simulink subsystem "ConfiguredSimscapePlantModels"  (R2022b)
settings: Solver=VariableStepAuto  StartTime=0.0  StopTime=10.0  RelTol=1e-3
undefined symbols (not defined in the file): AxlFL, AxlFR, AxlRL, AxlRR, EM1, EM2, PlntDCDCVoltInit, PlntDiffrntl2Axl1Damp, PlntDiffrntl2CarrDamp, PlntDiffrntl2Eff, PlntDiffrntl2PwrThresh, PlntDiffrntlAxl1Damp, PlntDiffrntlCarrDamp, PlntDiffrntlEff, PlntDiffrntlPwrThresh, PlntTrnsfrCaseAxlSpdLock, PlntTrnsfrCaseTrqSplitRatio
libraries: fl_lib x14, nesl_utility_internal x10, sdl_lib x5, nesl_utility x1
(part 1 of 2)
settings Model: ModifiedByFormat=The MathWorks, Inc.  Creator=The MathWorks, Inc.  LastModifiedBy=The MathWorks, Inc.
settings SolverCC: MaxZcPerStep=1
settings DebuggingCC: UnconnectedInputMsg=warning  UnconnectedOutputMsg=warning  UnconnectedLineMsg=warning
settings ModelReferenceCC: EnableRefExpFcnMdlSchedulingChecks=on
settings RTWCC: DLArmComputeVersion=19.05

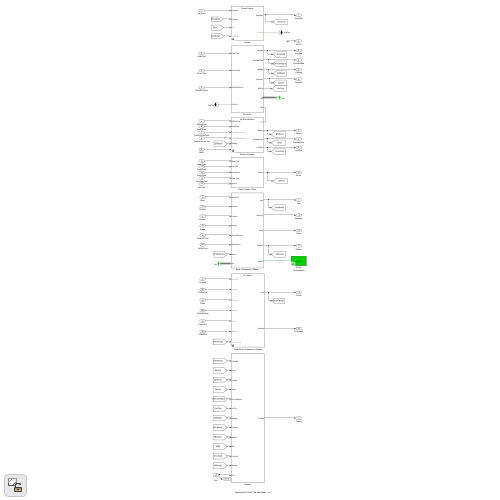
[thumbnail: Simulink's stored preview of the top-level diagram]
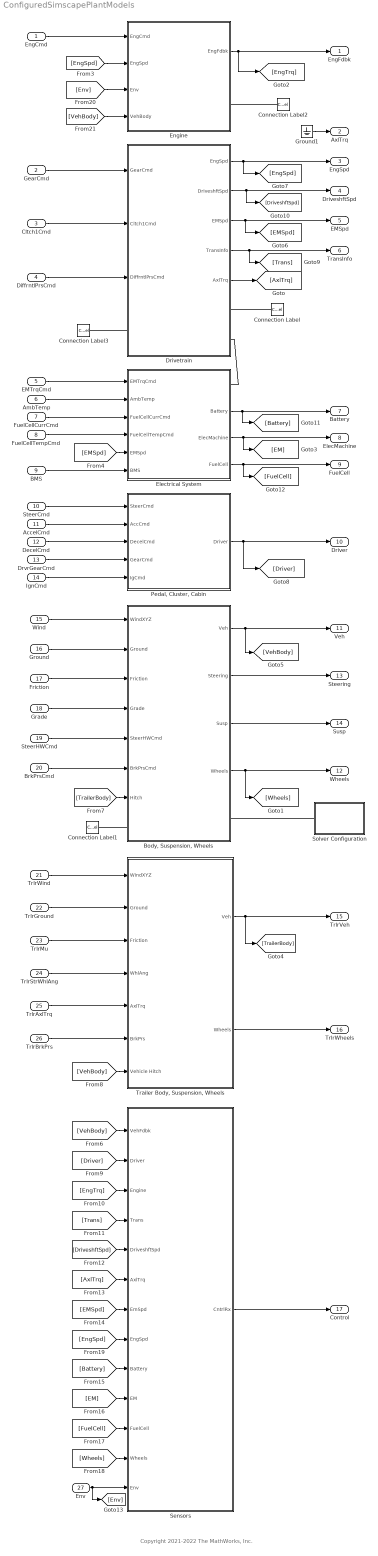
== system ConfiguredSimscapePlantModels ==
  note: Copyright 2021-2022 The MathWorks, Inc.
  EngCmd : Inport
  GearCmd : Inport  Port=2
  Cltch1Cmd : Inport  Port=3
  DiffrntlPrsCmd : Inport  Port=4
  EMTrqCmd : Inport  Port=5
  AmbTemp : Inport  Port=6
  FuelCellCurrCmd : Inport  Port=7
  FuelCellTempCmd : Inport  Port=8
  BMS : Inport  Port=9
  SteerCmd : Inport  Port=10
  AccelCmd : Inport  Port=11
  DecelCmd : Inport  Port=12
  DrvrGearCmd : Inport  Port=13
  IgnCmd : Inport  Port=14
  Wind : Inport  Port=15
  Ground : Inport  Port=16
  Friction : Inport  Port=17
  Grade : Inport  Port=18
  SteerHWCmd : Inport  Port=19
  BrkPrsCmd : Inport  Port=20
  TrlrWind : Inport  Port=21
  TrlrGround : Inport  Port=22
  TrlrMu : Inport  Port=23
  TrlrStrWhlAng : Inport  Port=24
  TrlrAxlTrq : Inport  Port=25
  TrlrBrkPrs : Inport  Port=26
  " Env" : Inport  Port=27
  "Body, Suspension, Wheels" : Subsystem  VariantControl=Longitudinal Vehicle Dynamics
  Connection Label : ConnectionLabel  Label=Axl
  Connection Label1 : ConnectionLabel  Label=Axl
  Connection Label2 : ConnectionLabel  Label=EngTrq
  Connection Label3 : ConnectionLabel  Label=EngTrq
  Drivetrain : Subsystem
  Electrical System : Subsystem  Variant=on  VariantControlMode=label  VariantControl=Choice  LabelModeActiveChoice=Electrical System 1EM
      settings: PortSchema="{\"entries\":[{\"content\":{\"sides\":[{\"content\":{\"connectorIds\":[\"In1\",\"In2\",\"In3\",\"In4\",\"In5\",\"In6\"]},\"type\":\"ConnectorPlacement.EquallySpacedRectSide\",\"uuid\":\"168fda7d-02fd-4045-80e4-d70d0b749a9c\"},{\"content\":{\"connectorIds\":[\"RConn1\",\"Out1\",\"Out2\",\"Out3\"],\"side\":\"RIGHT\"},\"type\":\"ConnectorPlacement.EquallySpacedRectSide\",\"uuid\":\"a7e9bf4a-b9ce-46d6-8afc-0075c6e03a0c\"},{\"content\":{\"connectorIds\":[],\"side\":\"TOP\"},\"type\":\"ConnectorPlacement.EquallySpacedRectSide\",\"uuid\":\"81c60468-d7ed-4851-a727-3a9a5b008640\"}]},\"type\":\"ConnectorPlacement.EquallySpacedConnector\",\"uuid\":\"8c7c8f28-264e-479c-b2d0-01b49dca4966\"}],\"packageUris\":[\"http://schema.mathworks.com/mf0/Connector/R2020b\"],\"version\":\"1.0\"}"
  Engine : Subsystem  Variant=on  VariantControlMode=label  LabelModeActiveChoice=No Engine
  Ground1 : Ground
  "Pedal, Cluster, Cabin" : Subsystem
  Sensors : Subsystem
  Solver Configuration : Subsystem  Variant=on  VariantControlMode=label  VariantControl=Choice  LabelModeActiveChoice=Solver Configuration
  "Trailer Body, Suspension, Wheels" : Subsystem  Variant=on  VariantControlMode=label  LabelModeActiveChoice=No Trailer
  EngFdbk : Outport
  AxlTrq : Outport  Port=2
  EngSpd : Outport  Port=3
  DriveshftSpd : Outport  Port=4
  EMSpd : Outport  Port=5
  TransInfo : Outport  Port=6
  Battery : Outport  Port=7
  ElecMachine : Outport  Port=8
  FuelCell : Outport  Port=9
  Driver : Outport  Port=10
  Veh : Outport  Port=11
  Wheels : Outport  Port=12
  Steering : Outport  Port=13
  Susp : Outport  Port=14
  TrlrVeh : Outport  Port=15
  TrlrWheels : Outport  Port=16
  Control : Outport  Port=17
  wires:
  Drivetrain/4(TransInfo) -> [Trans], TransInfo/1
  EngCmd/1 -> Engine/1(EngCmd)
  Electrical System/3(FuelCell) -> FuelCell/1, [FuelCell]
  Electrical System/1(Battery) -> Battery/1, [Battery]
  TrlrGround/1 -> "Trailer Body, Suspension, Wheels"/2(Ground)
  Wind/1 -> "Body, Suspension, Wheels"/1(WindXYZ)
  TrlrAxlTrq/1 -> "Trailer Body, Suspension, Wheels"/5(AxlTrq)
  EMTrqCmd/1 -> Electrical System/1(EMTrqCmd)
  DiffrntlPrsCmd/1 -> Drivetrain/3(DiffrntlPrsCmd)
  TrlrMu/1 -> "Trailer Body, Suspension, Wheels"/3(Friction)
  Friction/1 -> "Body, Suspension, Wheels"/3(Friction)
  SteerHWCmd/1 -> "Body, Suspension, Wheels"/5(SteerHWCmd)
  [EMSpd] -> Electrical System/5(EMSpd)
  Ground/1 -> "Body, Suspension, Wheels"/2(Ground)
  AmbTemp/1 -> Electrical System/2(AmbTemp)
  SteerCmd/1 -> "Pedal, Cluster, Cabin"/1(SteerCmd)
  TrlrBrkPrs/1 -> "Trailer Body, Suspension, Wheels"/6(BrkPrs)
  Drivetrain/2(DriveshftSpd) -> [DriveshftSpd], DriveshftSpd/1
  "Body, Suspension, Wheels"/1(Veh) -> [VehBody], Veh/1
  Engine/1(EngFdbk) -> [EngTrq], EngFdbk/1
  BrkPrsCmd/1 -> "Body, Suspension, Wheels"/6(BrkPrsCmd)
  Cltch1Cmd/1 -> Drivetrain/2(Cltch1Cmd)
  TrlrWind/1 -> "Trailer Body, Suspension, Wheels"/1(WindXYZ)
  TrlrStrWhlAng/1 -> "Trailer Body, Suspension, Wheels"/4(WhlAng)
  [VehBody] -> "Trailer Body, Suspension, Wheels"/7(Vehicle Hitch)
  "Trailer Body, Suspension, Wheels"/2(Wheels) -> TrlrWheels/1
  Electrical System/2(ElecMachine) -> [EM], ElecMachine/1
  [TrailerBody] -> "Body, Suspension, Wheels"/7(Hitch)
  DecelCmd/1 -> "Pedal, Cluster, Cabin"/3(DecelCmd)
  DrvrGearCmd/1 -> "Pedal, Cluster, Cabin"/4(GearCmd)
  Drivetrain/3(EMSpd) -> [EMSpd], EMSpd/1
  IgnCmd/1 -> "Pedal, Cluster, Cabin"/5(IgCmd)
  FuelCellTempCmd/1 -> Electrical System/4(FuelCellTempCmd)
  "Body, Suspension, Wheels"/2(Steering) -> Steering/1
  GearCmd/1 -> Drivetrain/1(GearCmd)
  "Body, Suspension, Wheels"/4(Wheels) -> [Wheels], Wheels/1
  "Trailer Body, Suspension, Wheels"/1(Veh) -> TrlrVeh/1, [TrailerBody]
  FuelCellCurrCmd/1 -> Electrical System/3(FuelCellCurrCmd)
  AccelCmd/1 -> "Pedal, Cluster, Cabin"/2(AccCmd)
  Drivetrain/1(EngSpd) -> EngSpd/1, [EngSpd]
  [VehBody] -> Sensors/1(VehFdbk)
  "Pedal, Cluster, Cabin"/1(Driver) -> Driver/1, [Driver]
  [Driver] -> Sensors/2(Driver)
  [EngTrq] -> Sensors/3(Engine)
  [Trans] -> Sensors/4(Trans)
  [DriveshftSpd] -> Sensors/5(DriveshftSpd)
  [AxlTrq] -> Sensors/6(AxlTrq)
  [EMSpd] -> Sensors/7(EmSpd)
  [Battery] -> Sensors/9(Battery)
  [EM] -> Sensors/10(EM)
  [FuelCell] -> Sensors/11(FuelCell)
  [Wheels] -> Sensors/12(Wheels)
  Sensors/1(CntrlRx) -> Control/1
  " Env"/1 -> Sensors/13(Env), [Env]
  [EngSpd] -> Sensors/8(EngSpd)
  [Env] -> Engine/3(Env)
  [VehBody] -> Engine/4(VehBody)
  [EngSpd] -> Engine/2(EngSpd)
  "Body, Suspension, Wheels"/3(Susp) -> Susp/1
  Grade/1 -> "Body, Suspension, Wheels"/4(Grade)
  Ground1/1 -> AxlTrq/1
  Drivetrain/5(AxlTrq) -> [AxlTrq]
  BMS/1 -> Electrical System/6(BMS)
  connections:
  Connection Label/LConn1 -- Drivetrain/RConn1
  "Body, Suspension, Wheels"/LConn1 -- Connection Label1/LConn1
  Electrical System/RConn1 -- Drivetrain/RConn2
  Drivetrain/LConn1 -- Connection Label3/LConn1
  Connection Label2/LConn1 -- Engine/RConn1
  Solver Configuration/RConn1 -- "Body, Suspension, Wheels"/RConn1

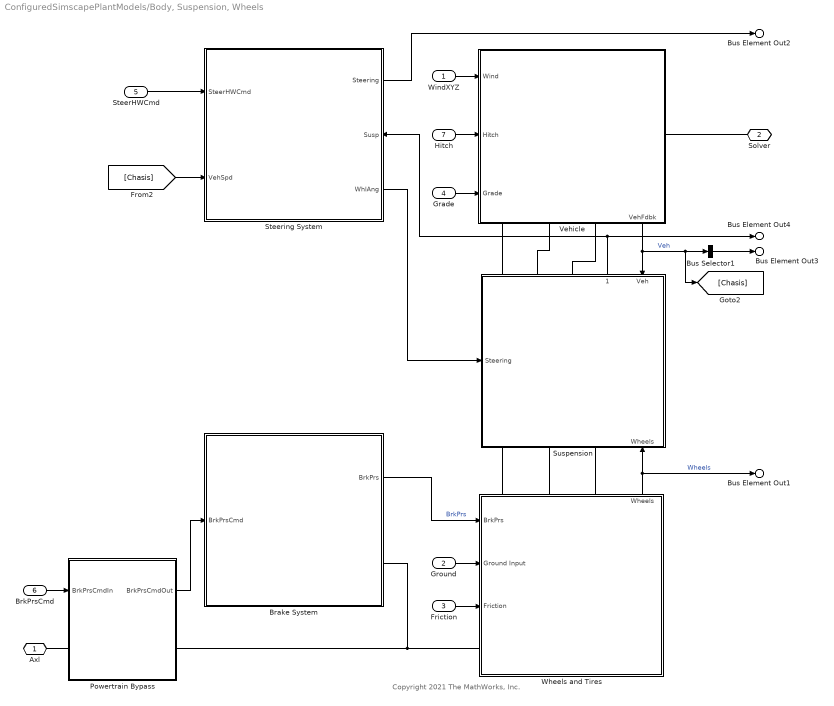
== system ConfiguredSimscapePlantModels/Body, Suspension, Wheels ==
  note: Copyright 2021 The MathWorks, Inc.
  WindXYZ : Inport  Unit=m/s  PortDimensions=3
  Ground : Inport  Port=2  Unit=m  PortDimensions=4
  Friction : Inport  Port=3  Unit=1  PortDimensions=4
  Grade : Inport  Port=4  Unit=deg  PortDimensions=1
  SteerHWCmd : Inport  Port=5  Unit=rad
  BrkPrsCmd : Inport  Port=6  PortDimensions=4
  Hitch : Inport  Port=7
  Brake System : Subsystem  Variant=on  VariantControlMode=label  VariantControl=Choice  LabelModeActiveChoice=Braking Hydraulics and Disc Brakes
      mask Display: disp('Brake System');
  Bus Selector1 : BusSelector  OutputSignals=InertFrm,BdyFrm  OutputAsBus=on
  Powertrain Bypass : Subsystem  Variant=on  VariantControlMode=label  VariantControl=Choice  LabelModeActiveChoice=Pass Through
  Steering System : Subsystem  Variant=on  VariantControlMode=label  VariantControl=0  LabelModeActiveChoice=No Steering
      settings: PortSchema="{\"entries\":[{\"content\":{\"sides\":[{\"content\":{\"connectorIds\":[\"In1\",\"In2\"]},\"type\":\"ConnectorPlacement.EquallySpacedRectSide\",\"uuid\":\"f4eae9a1-ee72-4894-9c3f-d81ee40fba89\"},{\"content\":{\"connectorIds\":[\"Out1\",\"In3\",\"Out2\"],\"side\":\"RIGHT\"},\"type\":\"ConnectorPlacement.EquallySpacedRectSide\",\"uuid\":\"c62a78d9-dc5d-4f96-a554-c82d7fa22a9e\"},{\"content\":{\"connectorIds\":[],\"side\":\"TOP\"},\"type\":\"ConnectorPlacement.EquallySpacedRectSide\",\"uuid\":\"38f3851a-1d1e-4a2b-8c09-8e5c8dcc7723\"}]},\"type\":\"ConnectorPlacement.EquallySpacedConnector\",\"uuid\":\"9f269846-92fa-4948-bc2b-71154f41fdde\"}],\"packageUris\":[\"http://schema.mathworks.com/mf0/Connector/R2020b\"],\"version\":\"1.0\"}"
      mask Display: disp('Steering System');
  Suspension : Subsystem  Variant=on  VariantControlMode=label  VariantControl=Choice  LabelModeActiveChoice=No Suspension
      settings: PortSchema="{\"entries\":[{\"content\":{\"sides\":[{\"content\":{\"connectorIds\":[\"In1\"]},\"type\":\"ConnectorPlacement.EquallySpacedRectSide\",\"uuid\":\"0a9265e3-f55e-4b74-9b74-681dc9522591\"},{\"content\":{\"connectorIds\":[],\"side\":\"RIGHT\"},\"type\":\"ConnectorPlacement.EquallySpacedRectSide\",\"uuid\":\"92df639a-7bc2-4e90-97ea-0cb216e2f16a\"},{\"content\":{\"connectorIds\":[\"LConn1\",\"LConn2\",\"LConn3\",\"Out1\",\"In2\"],\"side\":\"TOP\"},\"type\":\"ConnectorPlacement.EquallySpacedRectSide\",\"uuid\":\"2064b6cb-c7a8-4cfb-82de-a07750d990cb\"},{\"content\":{\"connectorIds\":[\"RConn1\",\"RConn2\",\"RConn3\",\"In3\"],\"side\":\"BOTTOM\"},\"type\":\"ConnectorPlacement.EquallySpacedRectSide\",\"uuid\":\"169bd4e6-c3fe-4e36-acea-c25875014463\"}]},\"type\":\"ConnectorPlacement.EquallySpacedConnector\",\"uuid\":\"e0b50182-0637-4594-80e7-4ddd0df85797\"}],\"packageUris\":[\"http://schema.mathworks.com/mf0/Connector/R2020b\"],\"version\":\"1.0\"}"
      mask Display: disp('Suspension');
  Vehicle : Subsystem  Variant=on  VariantControlMode=label  VariantControl=Choice  LabelModeActiveChoice=Vehicle Body 1DOF Longitudinal
      settings: PortSchema="{\"entries\":[{\"content\":{\"sides\":[{\"content\":{\"connectorIds\":[\"In1\",\"In2\",\"In3\"]},\"type\":\"ConnectorPlacement.EquallySpacedRectSide\",\"uuid\":\"0a9265e3-f55e-4b74-9b74-681dc9522591\"},{\"content\":{\"connectorIds\":[\"RConn1\"],\"side\":\"RIGHT\"},\"type\":\"ConnectorPlacement.EquallySpacedRectSide\",\"uuid\":\"92df639a-7bc2-4e90-97ea-0cb216e2f16a\"},{\"content\":{\"connectorIds\":[],\"side\":\"TOP\"},\"type\":\"ConnectorPlacement.EquallySpacedRectSide\",\"uuid\":\"2064b6cb-c7a8-4cfb-82de-a07750d990cb\"},{\"content\":{\"connectorIds\":[\"RConn2\",\"RConn3\",\"RConn4\",\"Out1\"],\"side\":\"BOTTOM\"},\"type\":\"ConnectorPlacement.EquallySpacedRectSide\",\"uuid\":\"2b34afca-0a88-43db-924f-6476183b84bd\"}]},\"type\":\"ConnectorPlacement.EquallySpacedConnector\",\"uuid\":\"e0b50182-0637-4594-80e7-4ddd0df85797\"}],\"packageUris\":[\"http://schema.mathworks.com/mf0/Connector/R2020b\"],\"version\":\"1.0\"}"
      mask Display: disp('Vehicle');
  Wheels and Tires : Subsystem  Variant=on  VariantControlMode=label  VariantControl=Choice  LabelModeActiveChoice=MF Tires Longitudinal
      settings: PortSchema="{\"entries\":[{\"content\":{\"sides\":[{\"content\":{\"connectorIds\":[\"In1\",\"In2\",\"In3\",\"LConn1\"]},\"type\":\"ConnectorPlacement.EquallySpacedRectSide\",\"uuid\":\"fdb4d4cd-d0c0-42d9-b073-775af31e96a1\"},{\"content\":{\"connectorIds\":[],\"side\":\"RIGHT\"},\"type\":\"ConnectorPlacement.EquallySpacedRectSide\",\"uuid\":\"04106ddf-9917-4cd4-b177-ae763d642686\"},{\"content\":{\"connectorIds\":[\"LConn2\",\"LConn3\",\"LConn4\",\"Out1\"],\"side\":\"TOP\"},\"type\":\"ConnectorPlacement.EquallySpacedRectSide\",\"uuid\":\"568bf95c-0e25-4c45-a134-c198357b75be\"}]},\"type\":\"ConnectorPlacement.EquallySpacedConnector\",\"uuid\":\"4f44df5e-0d14-43ea-934e-2abe86546e95\"}],\"packageUris\":[\"http://schema.mathworks.com/mf0/Connector/R2020b\"],\"version\":\"1.0\"}"
      mask Display: disp('Suspension');
  Axl : PMIOPort  Side=Left
  Solver : PMIOPort  Port=2  Side=Right
  Bus Element Out3 : Outport  PortName=Veh
  Bus Element Out2 : Outport  Port=2  PortName=Steering
  Bus Element Out4 : Outport  Port=3  PortName=Susp
  Bus Element Out1 : Outport  Port=4  PortName=Wheels
  wires:
  SteerHWCmd/1 -> Steering System/1(SteerHWCmd)
  Bus Selector1/1 -> Bus Element Out3/1
  WindXYZ/1 -> Vehicle/1(Wind)
  Brake System/1(BrkPrs) -> Wheels and Tires/1(BrkPrs)  "BrkPrs"
  Steering System/2(WhlAng) -> Suspension/1(Steering)
  Suspension/1(SuspChassis) -> Steering System/3(Susp), Bus Element Out4/1
  Powertrain Bypass/1(BrkPrsCmdOut) -> Brake System/1(BrkPrsCmd)
  Wheels and Tires/1(Wheels) -> Bus Element Out1/1, Suspension/3(Wheels)  "Wheels"
  Grade/1 -> Vehicle/3(Grade)
  Hitch/1 -> Vehicle/2(Hitch)
  Friction/1 -> Wheels and Tires/3(Friction)
  Steering System/1(Steering) -> Bus Element Out2/1
  [Chasis] -> Steering System/2(VehSpd)
  Ground/1 -> Wheels and Tires/2(Ground Input)
  Vehicle/1(VehFdbk) -> [Chasis], Bus Selector1/1, Suspension/2(Veh)  "Veh"
  BrkPrsCmd/1 -> Powertrain Bypass/1(BrkPrsCmdIn)
  connections:
  Brake System/RConn1 -- Powertrain Bypass/RConn1 -- Wheels and Tires/LConn1
  Vehicle/RConn2 -- Suspension/LConn1
  Vehicle/RConn3 -- Suspension/LConn2
  Vehicle/RConn4 -- Suspension/LConn3
  Wheels and Tires/LConn2 -- Suspension/RConn1
  Wheels and Tires/LConn3 -- Suspension/RConn2
  Wheels and Tires/LConn4 -- Suspension/RConn3
  Vehicle/RConn1 -- Solver/RConn1
  Axl/RConn1 -- Powertrain Bypass/LConn1

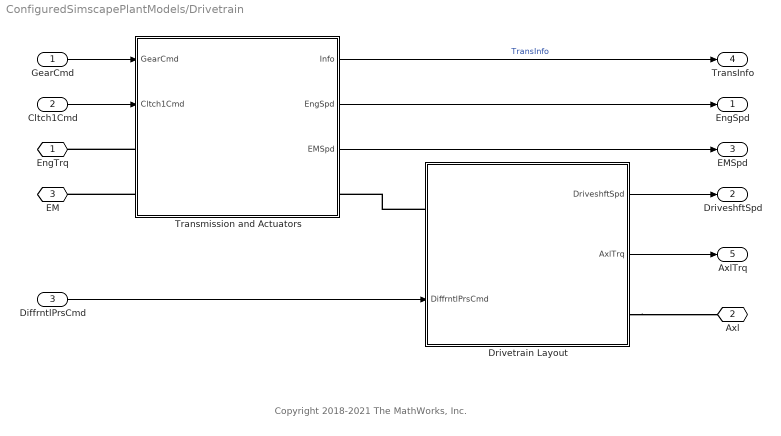
== system ConfiguredSimscapePlantModels/Drivetrain ==
  note: Copyright 2018-2021 The MathWorks, Inc.
  GearCmd : Inport
  Cltch1Cmd : Inport  Port=2
  DiffrntlPrsCmd : Inport  Port=3
  Drivetrain Layout : Subsystem  VariantControl=New
      settings: PortSchema="{\"entries\":[{\"content\":{\"sides\":[{\"content\":{\"connectorIds\":[\"LConn1\",\"In1\"]},\"type\":\"ConnectorPlacement.EquallySpacedRectSide\",\"uuid\":\"aca18566-8f68-4dbe-a1ea-7891e9b0f8a0\"},{\"content\":{\"connectorIds\":[\"Out1\",\"Out2\",\"RConn1\"],\"side\":\"RIGHT\"},\"type\":\"ConnectorPlacement.EquallySpacedRectSide\",\"uuid\":\"80817b32-8ae2-43ef-bc82-fae1c7a772cb\"},{\"content\":{\"connectorIds\":[],\"side\":\"TOP\"},\"type\":\"ConnectorPlacement.EquallySpacedRectSide\",\"uuid\":\"fadb27fa-7a73-4d3f-b69d-888e371ed2d5\"}]},\"type\":\"ConnectorPlacement.EquallySpacedConnector\",\"uuid\":\"7287b0c1-67df-44d5-bf90-b5b5a04fa161\"}],\"packageUris\":[\"http://schema.mathworks.com/mf0/Connector/R2020b\"],\"version\":\"1.0\"}"
  Transmission and Actuators : Subsystem  Variant=on  VariantControlMode=label  LabelModeActiveChoice=Electric Vehicle 1EM
  EngTrq : PMIOPort  Side=Left
  Axl : PMIOPort  Port=2  Side=Right
  EM : PMIOPort  Port=3  Side=Right
  EngSpd : Outport  Unit=rad/s  VectorParamsAs1DForOutWhenUnconnected=off
  DriveshftSpd : Outport  Port=2  VectorParamsAs1DForOutWhenUnconnected=off
  EMSpd : Outport  Port=3  Unit=rad/s  VectorParamsAs1DForOutWhenUnconnected=off
  TransInfo : Outport  Port=4  VectorParamsAs1DForOutWhenUnconnected=off
  AxlTrq : Outport  Port=5  VectorParamsAs1DForOutWhenUnconnected=off
  wires:
  Transmission and Actuators/1(Info) -> TransInfo/1  "TransInfo"
  DiffrntlPrsCmd/1 -> Drivetrain Layout/1(DiffrntlPrsCmd)
  Cltch1Cmd/1 -> Transmission and Actuators/2(Cltch1Cmd)
  Drivetrain Layout/1(DriveshftSpd) -> DriveshftSpd/1
  GearCmd/1 -> Transmission and Actuators/1(GearCmd)
  Transmission and Actuators/2(EngSpd) -> EngSpd/1
  Transmission and Actuators/3(EMSpd) -> EMSpd/1
  Drivetrain Layout/2(AxlTrq) -> AxlTrq/1
  connections:
  Transmission and Actuators/LConn2 -- EM/RConn1
  Drivetrain Layout/RConn1 -- Axl/RConn1
  Drivetrain Layout/LConn1 -- Transmission and Actuators/RConn1
  Transmission and Actuators/LConn1 -- EngTrq/RConn1

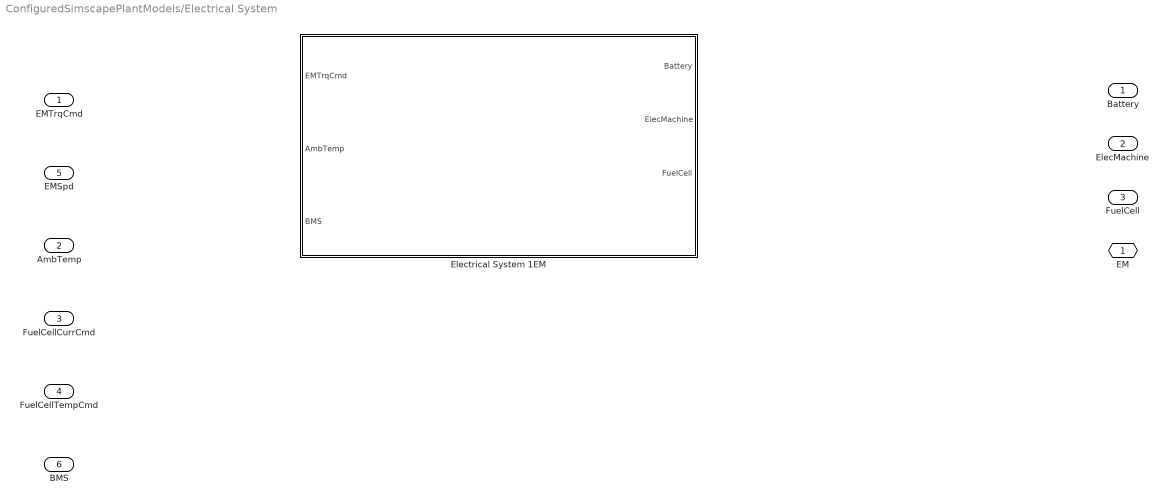
== system ConfiguredSimscapePlantModels/Electrical System ==
  EMTrqCmd : Inport
  AmbTemp : Inport  Port=2
  FuelCellCurrCmd : Inport  Port=3
  FuelCellTempCmd : Inport  Port=4
  EMSpd : Inport  Port=5
  BMS : Inport  Port=6
  Electrical System 1EM : Subsystem  VariantControl=Electrical System 1EM
  EM : PMIOPort  Side=Right
  Battery : Outport
  ElecMachine : Outport  Port=2
  FuelCell : Outport  Port=3

== system ConfiguredSimscapePlantModels/Engine ==
  EngCmd : Inport
  EngSpd : Inport  Port=2
  Env : Inport  Port=3
  VehBody : Inport  Port=4
  No Engine : Subsystem  VariantControl=No Engine  ReferencedSubsystem=NoEngine
  EngTrq : PMIOPort  Side=Right
  EngFdbk : Outport  VectorParamsAs1DForOutWhenUnconnected=off

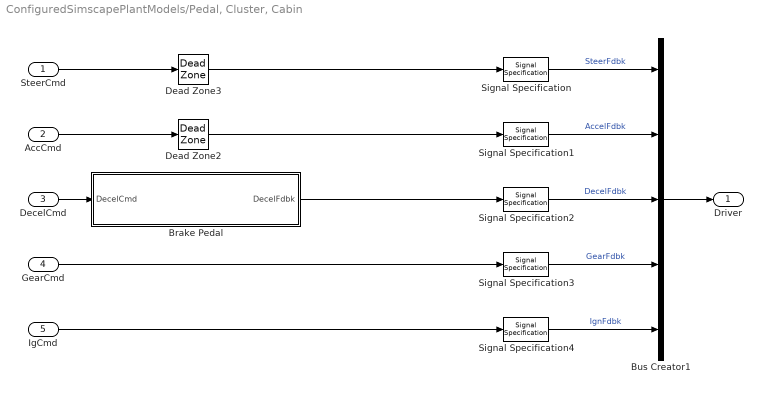
== system ConfiguredSimscapePlantModels/Pedal, Cluster, Cabin ==
  SteerCmd : Inport
  AccCmd : Inport  Port=2
  DecelCmd : Inport  Port=3
  GearCmd : Inport  Port=4
  IgCmd : Inport  Port=5
  Brake Pedal : Subsystem
  Bus Creator1 : BusCreator  Inputs=5
  Dead Zone2 : DeadZone  LowerValue=0  UpperValue=.01  ZeroCross=off
  Dead Zone3 : DeadZone  LowerValue=-.01  UpperValue=.01  ZeroCross=off
  Signal Specification : SignalSpecification  Unit=rad
  Signal Specification{1..4} (4 alike) : SignalSpecification  Unit=1
  Driver : Outport
  wires:
  Dead Zone3/1 -> Signal Specification/1
  Signal Specification1/1 -> Bus Creator1/2  "AccelFdbk"
  Signal Specification4/1 -> Bus Creator1/5  "IgnFdbk"
  Brake Pedal/1(DecelFdbk) -> Signal Specification2/1
  Signal Specification/1 -> Bus Creator1/1  "SteerFdbk"
  Signal Specification2/1 -> Bus Creator1/3  "DecelFdbk"
  GearCmd/1 -> Signal Specification3/1
  Bus Creator1/1 -> Driver/1
  IgCmd/1 -> Signal Specification4/1
  Signal Specification3/1 -> Bus Creator1/4  "GearFdbk"
  Dead Zone2/1 -> Signal Specification1/1
  SteerCmd/1 -> Dead Zone3/1
  AccCmd/1 -> Dead Zone2/1
  DecelCmd/1 -> Brake Pedal/1(DecelCmd)

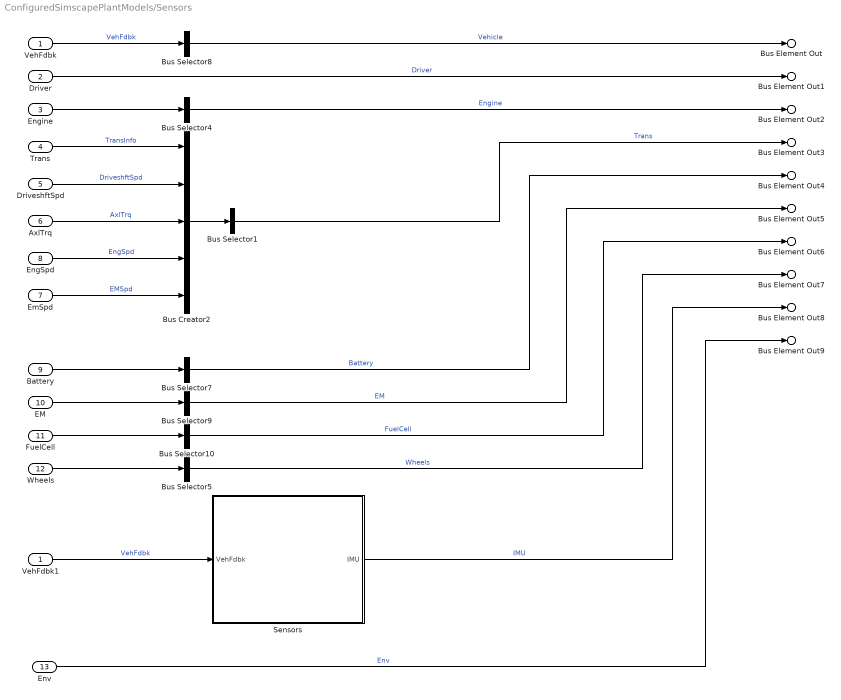
== system ConfiguredSimscapePlantModels/Sensors ==
  VehFdbk : Inport
  Driver : Inport  Port=2
  Engine : Inport  Port=3
  Trans : Inport  Port=4
  DriveshftSpd : Inport  Port=5
  AxlTrq : Inport  Port=6
  EmSpd : Inport  Port=7
  EngSpd : Inport  Port=8
  Battery : Inport  Port=9
  EM : Inport  Port=10
  FuelCell : Inport  Port=11
  Wheels : Inport  Port=12
  Env : Inport  Port=13
  Bus Creator2 : BusCreator  Inputs=5
  Bus Selector1 : BusSelector  OutputSignals=TransInfo.Cltch1State,TransInfo.Cltch2State,DriveshftSpd,AxlTrq,EngSpd,EMSpd,TransInfo.TransInfo.Trans.TransGear  OutputAsBus=on
  Bus Selector10 : BusSelector  OutputSignals=FuelCellVolt,FuelCellCurr,H2Flw  OutputAsBus=on
  Bus Selector4 : BusSelector  OutputSignals=EngTrq,Map,Mat,ThrPosPct,WgAreaPct,IntkCamPhase,ExhCamPhase,TurboRackPos,EgrVlvAreaPct,VarCompRatioPos,IntkVlvLift,VarIntkRunLen,Afr,IntkSwirlVlvPos,TurboSpd,Iat,Ect,EgrVlvDeltaPrs,EgrVlvInTemp  OutputAsBus=on
  Bus Selector5 : BusSelector  OutputSignals=Wheels.BrkPrs,Wheels.Kappa,Wheels.Alpha,Wheels.Omega  OutputAsBus=on
  Bus Selector7 : BusSelector  OutputSignals=BattSoc,BattVolt,BattCurr,BattPwr,BMSSensors  OutputAsBus=on
  Bus Selector8 : BusSelector  OutputSignals=BdyFrm.Cg.Vel.xdot  OutputAsBus=on
  Bus Selector9 : BusSelector  OutputSignals=EMTrq,EMPwrElec  OutputAsBus=on
  Sensors : Subsystem  Variant=on  VariantControlMode=label  VariantControl=Choice  LabelModeActiveChoice=No IMU Sensor
  VehFdbk1 : InportShadow
  Bus Element Out : Outport  PortName=CntrlRx  Element=Vehicle
  Bus Element Out1 : Outport  PortName=CntrlRx  Element=Driver
  Bus Element Out2 : Outport  PortName=CntrlRx  Element=Engine
  Bus Element Out3 : Outport  PortName=CntrlRx  Element=Trans
  Bus Element Out4 : Outport  PortName=CntrlRx  Element=Battery
  Bus Element Out5 : Outport  PortName=CntrlRx  Element=EM
  Bus Element Out6 : Outport  PortName=CntrlRx  Element=FuelCell
  Bus Element Out7 : Outport  PortName=CntrlRx  Element=Wheels
  Bus Element Out8 : Outport  PortName=CntrlRx  Element=IMU
  Bus Element Out9 : Outport  PortName=CntrlRx  Element=Env
  wires:
  Bus Selector1/1 -> Bus Element Out3/1  "Trans"
  Bus Creator2/1 -> Bus Selector1/1
  Trans/1 -> Bus Creator2/1  "TransInfo"
  EngSpd/1 -> Bus Creator2/4  "EngSpd"
  Env/1 -> Bus Element Out9/1  "Env"
  Driver/1 -> Bus Element Out1/1  "Driver"
  Sensors/1(IMU) -> Bus Element Out8/1  "IMU"
  VehFdbk1/1 -> Sensors/1(VehFdbk)  "VehFdbk"
  Wheels/1 -> Bus Selector5/1
  FuelCell/1 -> Bus Selector10/1
  EM/1 -> Bus Selector9/1
  Battery/1 -> Bus Selector7/1
  EmSpd/1 -> Bus Creator2/5  "EMSpd"
  AxlTrq/1 -> Bus Creator2/3  "AxlTrq"
  DriveshftSpd/1 -> Bus Creator2/2  "DriveshftSpd"
  Engine/1 -> Bus Selector4/1
  VehFdbk/1 -> Bus Selector8/1  "VehFdbk"
  Bus Selector4/1 -> Bus Element Out2/1  "Engine"
  Bus Selector10/1 -> Bus Element Out6/1  "FuelCell"
  Bus Selector9/1 -> Bus Element Out5/1  "EM"
  Bus Selector8/1 -> Bus Element Out/1  "Vehicle"
  Bus Selector7/1 -> Bus Element Out4/1  "Battery"
  Bus Selector5/1 -> Bus Element Out7/1  "Wheels"

== system ConfiguredSimscapePlantModels/Solver Configuration ==
  Solver Configuration : nesl_utility/Solver Configuration  VariantControl=Solver Configuration  PhysicalDomain=network_engine_domain  SubClassName=solver  LeftPortType=input  RightPortType=generic  Tones=[]  Harmonics=[]  SimulateNoise=off  Profile=off  UseLocalSampling=off  EnableSwitchedLinearOptims=on  FrequencyDomain=off  UseCCode=off  RelTol=0.001  AbsTol=0.001  MinStep=1e-09  ToWorkspace=off  RevertToSquareIcSolve=off  NumHomotopyIterations=100  PhasorMode=off  PhasorModeNumHarmonics=1  ConsistencySolver=NEWTON_XTOL_AFTER_FTOL  IndexReductionMethod=DerivativeReplacement  DoDC=off  ResidualTolerance=1e-09  ConsistencyTolSource=LOCAL  ConsistencyAbsTol=0.001  ConsistencyRelTol=0.001  ConsistencyTolFactor=0.001  UseLocalSolver=off  LocalSolverChoice=NE_BACKWARD_EULER_ADVANCER  ResolveIndetEquations=on  FunctionEvalNumThread=1  LocalSolverSampleTime=0.001  DoFixedCost=off  MaxNonlinIter=3  MaxModeIter=2  ComputeImpulses=off  ImpulseIterations=2  LinearAlgebra=auto  LinearAlgebraNumThread=0  EquationFormulation=NE_TIME_EF  DelaysMemoryBudget=1024  AutomaticFiltering=on  FilteringTimeConstant=0.001  PartitionStorageMethod=AS_NEEDED  PartitionMemoryBudget=1024  PartitionMethod=ROBUST
  a : PMIOPort  Side=Right

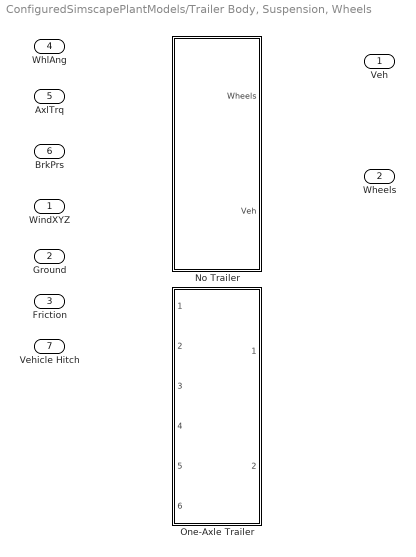
== system ConfiguredSimscapePlantModels/Trailer Body, Suspension, Wheels ==
  WindXYZ : Inport
  Ground : Inport  Port=2
  Friction : Inport  Port=3
  WhlAng : Inport  Port=4
  AxlTrq : Inport  Port=5
  BrkPrs : Inport  Port=6
  Vehicle Hitch : Inport  Port=7
  No Trailer : Subsystem  VariantControl=No Trailer
  One-Axle Trailer : Subsystem  VariantControl=One-Axle Trailer  ReferencedSubsystem=OneAxleTrailer
  Veh : Outport  VectorParamsAs1DForOutWhenUnconnected=off
  Wheels : Outport  Port=2  VectorParamsAs1DForOutWhenUnconnected=off

== system ConfiguredSimscapePlantModels/Body, Suspension, Wheels/Brake System ==
  BrkPrsCmd : Inport
  Braking Hydraulics and Disc Brakes : Subsystem  VariantControl=Braking Hydraulics and Disc Brakes  ReferencedSubsystem=BrakingHydraulicsDiscBrakesSSC
  Axl : PMIOPort  Side=Right
  BrkPrs : Outport

== system ConfiguredSimscapePlantModels/Body, Suspension, Wheels/Powertrain Bypass ==
  BrkPrsCmdIn : Inport
  External Signal Source : Subsystem  VariantControl=External Signal Source
  Pass Through : Subsystem  VariantControl=Pass Through
  AxlTrqIn : PMIOPort  Side=Left
  AxlTrqOut : PMIOPort  Port=2  Side=Right
  BrkPrsCmdOut : Outport

== system ConfiguredSimscapePlantModels/Body, Suspension, Wheels/Steering System ==
  SteerHWCmd : Inport
  VehSpd : Inport  Port=2
  Susp : Inport  Port=3
  No Steering : Subsystem  VariantControl=No Steering  ReferencedSubsystem=NoSteering
  Steering : Outport
  WhlAng : Outport  Port=2  VectorParamsAs1DForOutWhenUnconnected=off

== system ConfiguredSimscapePlantModels/Body, Suspension, Wheels/Suspension ==
  Steering : Inport
  Veh : Inport  Port=2
  Wheels : Inport  Port=3
  No Suspension : Subsystem  VariantControl=No Suspension  ReferencedSubsystem=NoSuspensionSSC
  Suspension : PMIOPort  Side=Left
  FzF : PMIOPort  Port=2  Side=Left
  FzR : PMIOPort  Port=3  Side=Left
  Suspension1 : PMIOPort  Port=4  Side=Right
  FzF1 : PMIOPort  Port=5  Side=Right
  FzR1 : PMIOPort  Port=6  Side=Right
  SuspChassis : Outport

== system ConfiguredSimscapePlantModels/Body, Suspension, Wheels/Vehicle ==
  Wind : Inport
  Hitch : Inport  Port=2
  Grade : Inport  Port=3
  Vehicle Body 1DOF Longitudinal : Subsystem  VariantControl=Vehicle Body 1DOF Longitudinal  ReferencedSubsystem=VehicleBody1DOFLongitudinalSSC
  Solver : PMIOPort  Side=Right
  Suspension : PMIOPort  Port=2  Side=Right
  FzF : PMIOPort  Port=3  Side=Right
  FzR : PMIOPort  Port=4  Side=Right
  VehFdbk : Outport

== system ConfiguredSimscapePlantModels/Body, Suspension, Wheels/Wheels and Tires ==
  BrkPrs : Inport
  Ground Input : Inport  Port=2
  Friction : Inport  Port=3
  MF Tires Longitudinal : Subsystem  VariantControl=MF Tires Longitudinal  ReferencedSubsystem=MFTiresLongitudinalSSC
  Axl : PMIOPort  Side=Left
  Suspension : PMIOPort  Port=2  Side=Left
  FzF : PMIOPort  Port=3  Side=Left
  FzR : PMIOPort  Port=4  Side=Left
  Wheels : Outport

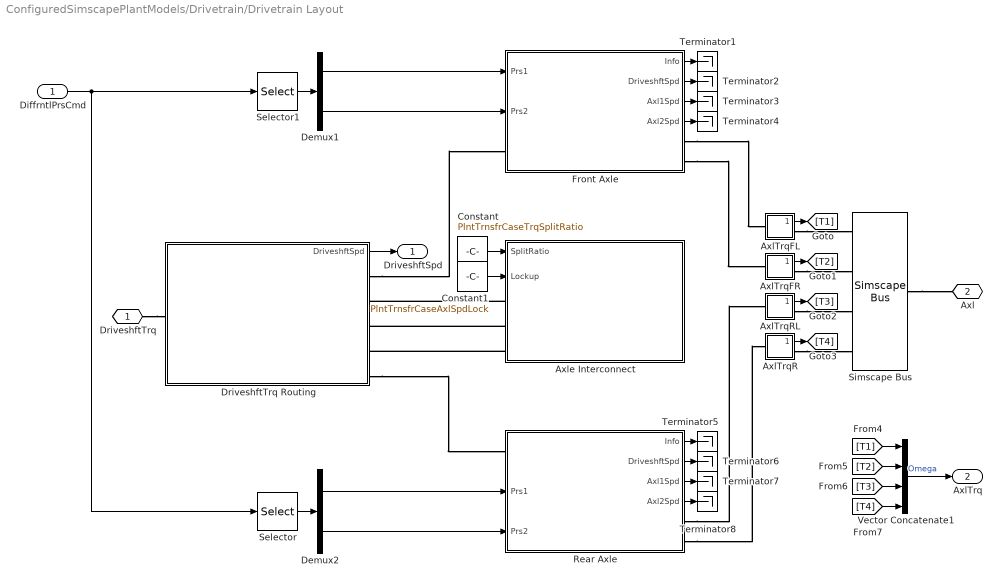
== system ConfiguredSimscapePlantModels/Drivetrain/Drivetrain Layout ==
  DiffrntlPrsCmd : Inport
  AxlTrqFL : Subsystem
  AxlTrqFR : Subsystem
  AxlTrqR : Subsystem
  AxlTrqRL : Subsystem
  Axle Interconnect : Subsystem  Variant=on  VariantControlMode=label  VariantControl=Choice  LabelModeActiveChoice=No Interconnect
  Constant : Constant  Value=PlntTrnsfrCaseTrqSplitRatio  SampleTime=-1
  Constant1 : Constant  Value=PlntTrnsfrCaseAxlSpdLock  SampleTime=-1
  Demux1 : Demux  Outputs=2
  Demux2 : Demux  Outputs=2
  DriveshftTrq Routing : Subsystem  Variant=on  VariantControlMode=label  VariantControl=Choice  LabelModeActiveChoice=Two Actuator AWD
  Front Axle : Subsystem  Variant=on  VariantControlMode=label  VariantControl=Choice  LabelModeActiveChoice=Open Differential
  Rear Axle : Subsystem  Variant=on  VariantControlMode=label  VariantControl=Choice  LabelModeActiveChoice=Open Differential
      settings: PortSchema="{\"entries\":[{\"content\":{\"sides\":[{\"content\":{\"connectorIds\":[\"LConn1\",\"In1\",\"In2\"]},\"type\":\"ConnectorPlacement.EquallySpacedRectSide\",\"uuid\":\"74f8b1d8-6b3a-4eeb-b984-715de40eb708\"},{\"content\":{\"connectorIds\":[\"Out1\",\"Out2\",\"Out3\",\"Out4\",\"RConn1\",\"RConn2\"],\"side\":\"RIGHT\"},\"type\":\"ConnectorPlacement.EquallySpacedRectSide\",\"uuid\":\"c00021b1-b8b4-4ff3-9b35-429da9caaad3\"},{\"content\":{\"connectorIds\":[],\"side\":\"TOP\"},\"type\":\"ConnectorPlacement.EquallySpacedRectSide\",\"uuid\":\"0bf4e327-a693-4202-b285-43d08d42df4d\"}]},\"type\":\"ConnectorPlacement.EquallySpacedConnector\",\"uuid\":\"b41f4b2c-0e15-48ba-ac2c-145a8c4b8844\"}],\"packageUris\":[\"http://schema.mathworks.com/mf0/Connector/R2020b\"],\"version\":\"1.0\"}"
  Selector : Selector  InputPortWidth=4  IndexOptions=Index vector (dialog)  Indices=[3 4]  OutputSizes=1
  Selector1 : Selector  InputPortWidth=4  IndexOptions=Index vector (dialog)  Indices=[1 2]  OutputSizes=1
  Simscape Bus : SimscapeBus  HierarchyStrings=AxlFL;AxlFR;AxlRL;AxlRR
  Terminator{1..8} (8 alike) : Terminator
  Vector Concatenate1 : Concatenate  NumInputs=4
  DriveshftTrq : PMIOPort  Side=Left
  Axl : PMIOPort  Port=2  Side=Right
  DriveshftSpd : Outport  VectorParamsAs1DForOutWhenUnconnected=off
  AxlTrq : Outport  Port=2  VectorParamsAs1DForOutWhenUnconnected=off
  wires:
  Selector/1 -> Demux2/1
  Demux1/2 -> Front Axle/2(Prs2)
  Demux1/1 -> Front Axle/1(Prs1)
  Selector1/1 -> Demux1/1
  DiffrntlPrsCmd/1 -> Selector1/1, Selector/1
  Rear Axle/1(Info) -> Terminator5/1
  Front Axle/1(Info) -> Terminator1/1
  Demux2/1 -> Rear Axle/1(Prs1)
  Demux2/2 -> Rear Axle/2(Prs2)
  Front Axle/2(DriveshftSpd) -> Terminator2/1
  Front Axle/3(Axl1Spd) -> Terminator3/1
  Front Axle/4(Axl2Spd) -> Terminator4/1
  Rear Axle/2(DriveshftSpd) -> Terminator6/1
  Rear Axle/3(Axl1Spd) -> Terminator7/1
  Rear Axle/4(Axl2Spd) -> Terminator8/1
  Constant/1 -> Axle Interconnect/1(SplitRatio)
  Constant1/1 -> Axle Interconnect/2(Lockup)
  [T4] -> Vector Concatenate1/4
  [T3] -> Vector Concatenate1/3
  [T2] -> Vector Concatenate1/2
  Vector Concatenate1/1 -> AxlTrq/1  "Omega"
  [T1] -> Vector Concatenate1/1
  AxlTrqFL/1(Trq) -> [T1]
  AxlTrqFR/1(Trq) -> [T2]
  AxlTrqRL/1(Trq) -> [T3]
  AxlTrqR/1(Trq) -> [T4]
  DriveshftTrq Routing/1(DriveshftSpd) -> DriveshftSpd/1
  connections:
  Simscape Bus/RConn1 -- Axl/RConn1
  Front Axle/RConn1 -- AxlTrqFL/LConn1
  Front Axle/RConn2 -- AxlTrqFR/LConn1
  Rear Axle/RConn2 -- AxlTrqR/LConn1
  Rear Axle/RConn1 -- AxlTrqRL/LConn1
  DriveshftTrq Routing/RConn1 -- Front Axle/LConn1
  DriveshftTrq Routing/RConn5 -- Rear Axle/LConn1
  Axle Interconnect/LConn1 -- DriveshftTrq Routing/RConn2
  Axle Interconnect/LConn2 -- DriveshftTrq Routing/RConn3
  Axle Interconnect/LConn3 -- DriveshftTrq Routing/RConn4
  AxlTrqFL/RConn1 -- Simscape Bus/LConn1
  AxlTrqFR/RConn1 -- Simscape Bus/LConn2
  AxlTrqRL/RConn1 -- Simscape Bus/LConn3
  AxlTrqR/RConn1 -- Simscape Bus/LConn4
  DriveshftTrq/RConn1 -- DriveshftTrq Routing/LConn1

== system ConfiguredSimscapePlantModels/Drivetrain/Transmission and Actuators ==
  GearCmd : Inport
  Cltch1Cmd : Inport  Port=2
  Electric Vehicle 1EM : Subsystem  VariantControl=Electric Vehicle 1EM  ReferencedSubsystem=BEV1EMSSC
  EngTrq : PMIOPort  Side=Left
  EM : PMIOPort  Port=2  Side=Left
  DriveshftTrq : PMIOPort  Port=3  Side=Right
  Info : Outport  VectorParamsAs1DForOutWhenUnconnected=off
  EngSpd : Outport  Port=2  VectorParamsAs1DForOutWhenUnconnected=off
  EMSpd : Outport  Port=3  VectorParamsAs1DForOutWhenUnconnected=off  BusOutputAsStruct=on

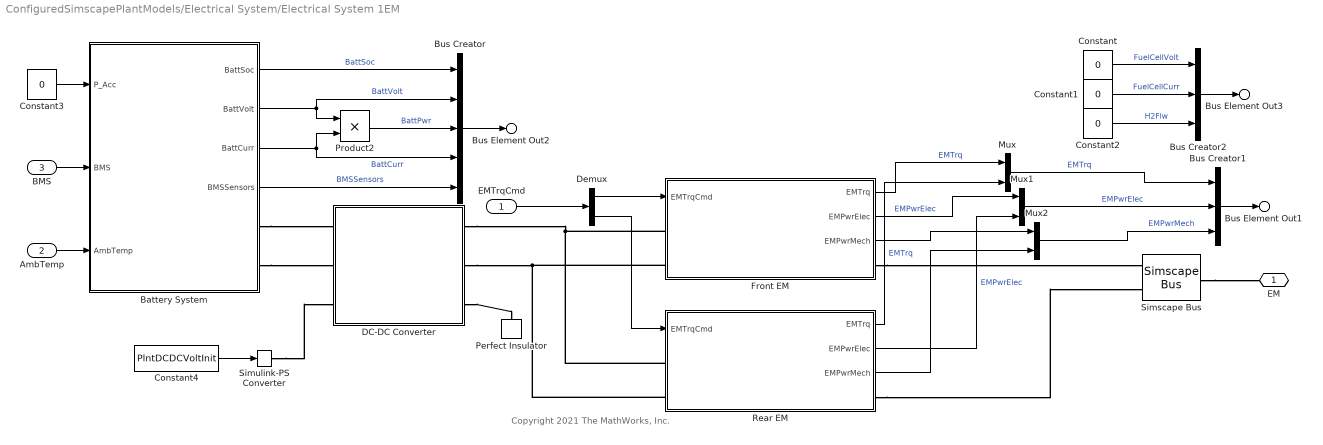
== system ConfiguredSimscapePlantModels/Electrical System/Electrical System 1EM ==
  note: Copyright 2021 The MathWorks, Inc.
  EMTrqCmd : Inport
  AmbTemp : Inport  Port=2
  BMS : Inport  Port=3
  Battery System : Subsystem  Variant=on  VariantControlMode=label  LabelModeActiveChoice=Mapped Battery
  Bus Creator : BusCreator  Inputs=5
  Bus Creator1 : BusCreator  Inputs=3
  Bus Creator2 : BusCreator  Inputs=3
  Constant{,1..3} (4 alike) : Constant  Value=0  SampleTime=-1
  Constant4 : Constant  Value=PlntDCDCVoltInit  SampleTime=-1
  DC-DC Converter : Subsystem  Variant=on  VariantControlMode=label  VariantControl=Choice  LabelModeActiveChoice=No DC-DC Converter
  Demux : Demux  Outputs=2
  Front EM : Subsystem
  Mux : Mux  Inputs=2
  Mux1 : Mux  Inputs=2
  Mux2 : Mux  Inputs=2
  Perfect Insulator : fl_lib/Thermal/Thermal Elements/Perfect Insulator  T_specify=off  T_priority=None  T=293.15 K  T_nominal_specify=off  T_nominal_unit=K  T_nominal_value=1
  Product2 : Product
  Rear EM : Subsystem
  Simscape Bus : SimscapeBus  HierarchyStrings=EM1;EM2
  Simulink-PS Converter : nesl_utility_internal/Simulink-PS Converter  PhysicalDomain=network_engine_domain  SubClassName=ps_input  LeftPortType=input  RightPortType=output  PseudoPeriodic=off  Frequencies=[]  NoiseDistribution=none  NoiseParameters=[]  Unit=1  AffineConversion=off  FilteringAndDerivatives=provide  SimscapeFilterOrder=1  InputFilterTimeConstant=0.001  UdotUserProvided=0
  EM : PMIOPort  Side=Right
  Bus Element Out2 : Outport  PortName=Battery
  Bus Element Out1 : Outport  Port=2  PortName=ElecMachine
  Bus Element Out3 : Outport  Port=3  PortName=FuelCell
  wires:
  Mux2/1 -> Bus Creator1/3  "EMPwrMech"
  Rear EM/3(EMPwrMech) -> Mux2/2
  Front EM/3(EMPwrMech) -> Mux2/1
  Mux1/1 -> Bus Creator1/2  "EMPwrElec"
  Rear EM/2(EMPwrElec) -> Mux1/2  "EMPwrElec"
  Front EM/2(EMPwrElec) -> Mux1/1  "EMPwrElec"
  Mux/1 -> Bus Creator1/1  "EMTrq"
  Rear EM/1(EMTrq) -> Mux/2  "EMTrq"
  Front EM/1(EMTrq) -> Mux/1  "EMTrq"
  Demux/2 -> Rear EM/1(EMTrqCmd)
  Demux/1 -> Front EM/1(EMTrqCmd)
  EMTrqCmd/1 -> Demux/1
  Constant3/1 -> Battery System/1(P_Acc)
  Constant/1 -> Bus Creator2/1  "FuelCellVolt"
  Bus Creator2/1 -> Bus Element Out3/1
  Bus Creator1/1 -> Bus Element Out1/1
  Constant2/1 -> Bus Creator2/3  "H2Flw"
  Constant1/1 -> Bus Creator2/2  "FuelCellCurr"
  Bus Creator/1 -> Bus Element Out2/1
  Battery System/2(BattVolt) -> Bus Creator/2, Product2/1  "BattVolt"
  Battery System/3(BattCurr) -> Bus Creator/4, Product2/2  "BattCurr"
  Battery System/1(BattSoc) -> Bus Creator/1  "BattSoc"
  Product2/1 -> Bus Creator/3  "BattPwr"
  Constant4/1 -> Simulink-PS Converter/1
  BMS/1 -> Battery System/2(BMS)
  AmbTemp/1 -> Battery System/3(AmbTemp)
  Battery System/4(BMSSensors) -> Bus Creator/5  "BMSSensors"
  connections:
  Rear EM/RConn1 -- Simscape Bus/LConn2
  Front EM/RConn1 -- Simscape Bus/LConn1
  Rear EM/LConn2 -- DC-DC Converter/RConn2 -- Front EM/LConn2
  Rear EM/LConn1 -- Front EM/LConn1 -- DC-DC Converter/RConn1
  DC-DC Converter/RConn3 -- Perfect Insulator/LConn1
  Simscape Bus/RConn1 -- EM/RConn1
  Simulink-PS Converter/RConn1 -- DC-DC Converter/LConn3
  Battery System/RConn1 -- DC-DC Converter/LConn1
  Battery System/RConn2 -- DC-DC Converter/LConn2

== system ConfiguredSimscapePlantModels/Pedal, Cluster, Cabin/Brake Pedal ==
  DecelCmd : Inport
  Dead Zone1 : DeadZone  Commented=through  LowerValue=0  UpperValue=.01  ZeroCross=off
  DecelFdbk : Outport
  wires:
  Dead Zone1/1 -> DecelFdbk/1
  DecelCmd/1 -> Dead Zone1/1

== system ConfiguredSimscapePlantModels/Sensors/Sensors ==
  VehFdbk : Inport
  No IMU Sensor : Subsystem  VariantControl=No IMU Sensor
  IMU : Outport

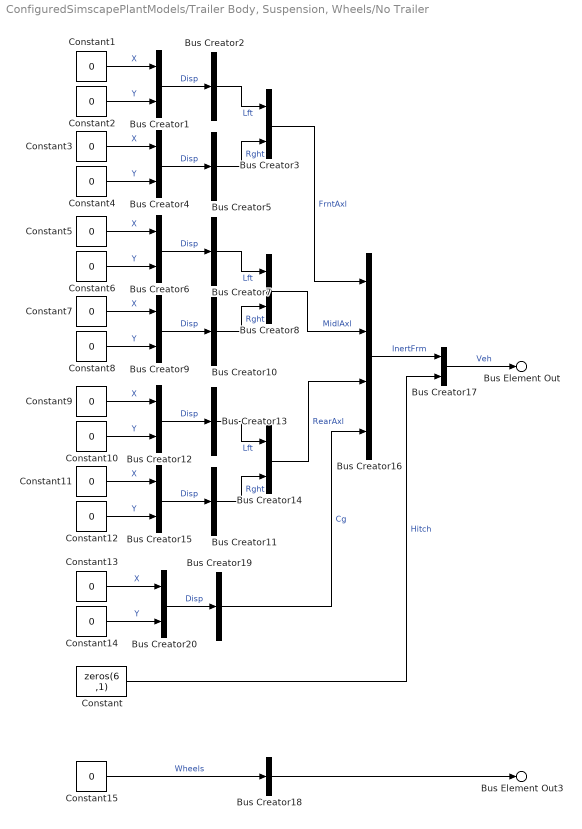
== system ConfiguredSimscapePlantModels/Trailer Body, Suspension, Wheels/No Trailer ==
  Bus Creator{1,3..4,6,8..9,12,14..15,17,20} (11 alike) : BusCreator  Inputs=2
  Bus Creator{2,5,7,10..11,13,18..19} (8 alike) : BusCreator  Inputs=1
  Bus Creator16 : BusCreator  Inputs=4
  Constant : Constant  Value=zeros(6 ,1)  SampleTime=-1
  Constant{1..15} (15 alike) : Constant  Value=0  SampleTime=-1
  Bus Element Out3 : Outport  PortName=Wheels
  Bus Element Out : Outport  Port=2  PortName=Veh
  wires:
  Constant1/1 -> Bus Creator1/1  "X"
  Bus Creator18/1 -> Bus Element Out3/1
  Constant2/1 -> Bus Creator1/2  "Y"
  Bus Creator1/1 -> Bus Creator2/1  "Disp"
  Bus Creator4/1 -> Bus Creator5/1  "Disp"
  Constant4/1 -> Bus Creator4/2  "Y"
  Constant3/1 -> Bus Creator4/1  "X"
  Bus Creator5/1 -> Bus Creator3/2  "Rght"
  Bus Creator2/1 -> Bus Creator3/1  "Lft"
  Bus Creator7/1 -> Bus Creator8/1  "Lft"
  Bus Creator10/1 -> Bus Creator8/2  "Rght"
  Constant7/1 -> Bus Creator9/1  "X"
  Constant8/1 -> Bus Creator9/2  "Y"
  Bus Creator9/1 -> Bus Creator10/1  "Disp"
  Bus Creator6/1 -> Bus Creator7/1  "Disp"
  Constant6/1 -> Bus Creator6/2  "Y"
  Constant5/1 -> Bus Creator6/1  "X"
  Constant9/1 -> Bus Creator12/1  "X"
  Constant10/1 -> Bus Creator12/2  "Y"
  Bus Creator12/1 -> Bus Creator13/1  "Disp"
  Bus Creator15/1 -> Bus Creator11/1  "Disp"
  Constant12/1 -> Bus Creator15/2  "Y"
  Constant11/1 -> Bus Creator15/1  "X"
  Bus Creator11/1 -> Bus Creator14/2  "Rght"
  Bus Creator13/1 -> Bus Creator14/1  "Lft"
  Bus Creator8/1 -> Bus Creator16/2  "MidlAxl"
  Bus Creator14/1 -> Bus Creator16/3  "RearAxl"
  Bus Creator3/1 -> Bus Creator16/1  "FrntAxl"
  Bus Creator16/1 -> Bus Creator17/1  "InertFrm"
  Bus Creator17/1 -> Bus Element Out/1  "Veh"
  Constant15/1 -> Bus Creator18/1  "Wheels"
  Bus Creator19/1 -> Bus Creator16/4  "Cg"
  Constant13/1 -> Bus Creator20/1  "X"
  Constant14/1 -> Bus Creator20/2  "Y"
  Bus Creator20/1 -> Bus Creator19/1  "Disp"
  Constant/1 -> Bus Creator17/2  "Hitch"

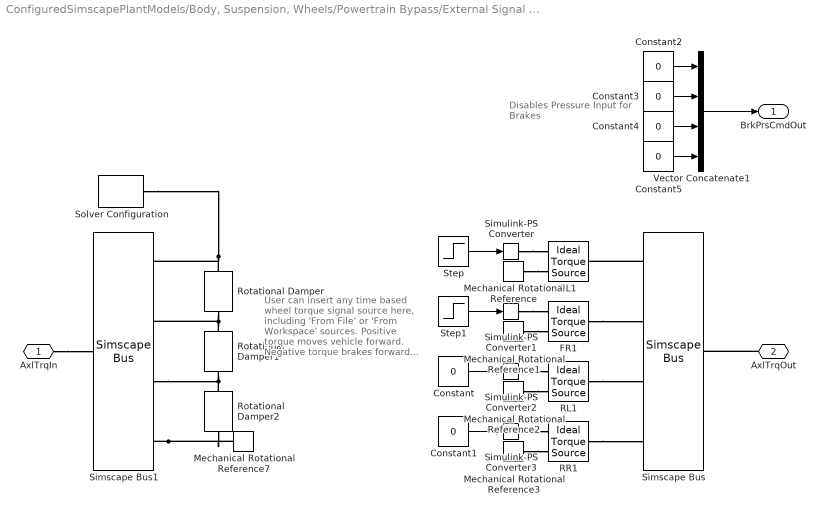
== system ConfiguredSimscapePlantModels/Body, Suspension, Wheels/Powertrain Bypass/External Signal Source ==
  note: User can insert any time based
      | wheel torque signal source here,
      | including 'From File' or 'From
      | Workspace' sources.
      |
      | Positive torque moves vehicle
      | forward.
      | Negative torque brakes forward
      | moving vehicle or moves vehicle
      | in reverse.
  note: Disables Pressure
      | Input for Brakes
  Constant{,1..5} (6 alike) : Constant  Value=0  SampleTime=-1
  FL1 : fl_lib/Mechanical/Mechanical Sources/Ideal Torque Source
  FR1 : fl_lib/Mechanical/Mechanical Sources/Ideal Torque Source
  Mechanical Rotational Reference{,1..3,7} (5 alike) : fl_lib/Mechanical/Rotational Elements/Mechanical Rotational Reference
  RL1 : fl_lib/Mechanical/Mechanical Sources/Ideal Torque Source
  RR1 : fl_lib/Mechanical/Mechanical Sources/Ideal Torque Source
  Rotational Damper : sdl_lib/Couplings & Drives/Springs & Dampers/Rotational Damper  D=1e5 N*m*s/rad  enable_faults=simscape.enum.onoff.off  b_fault=100 N*m*s/rad  temporal_fault=simscape.enum.onoff.off  fault_time=5 s  shock_fault=simscape.enum.onoff.off  acceleration_limit=100 rad/s^2  shock_limit=1  report_fault=simscape.enum.assert.action.none  thermal_port=simscape.enum.thermaleffects.omit  thermal_mass=50 kJ/K  temperature_specify=off  temperature_priority=High  temperature=300 K  temperature_nominal_specify=off  temperature_nominal_unit=K  temperature_nominal_value=1
  Rotational Damper1 : sdl_lib/Couplings & Drives/Springs & Dampers/Rotational Damper  D=1e5 N*m*s/rad  enable_faults=simscape.enum.onoff.off  b_fault=100 N*m*s/rad  temporal_fault=simscape.enum.onoff.off  fault_time=5 s  shock_fault=simscape.enum.onoff.off  acceleration_limit=100 rad/s^2  shock_limit=1  report_fault=simscape.enum.assert.action.none  thermal_port=simscape.enum.thermaleffects.omit  thermal_mass=50 kJ/K  temperature_specify=off  temperature_priority=High  temperature=300 K  temperature_nominal_specify=off  temperature_nominal_unit=K  temperature_nominal_value=1
  Rotational Damper2 : sdl_lib/Couplings & Drives/Springs & Dampers/Rotational Damper  D=1e5 N*m*s/rad  enable_faults=simscape.enum.onoff.off  b_fault=100 N*m*s/rad  temporal_fault=simscape.enum.onoff.off  fault_time=5 s  shock_fault=simscape.enum.onoff.off  acceleration_limit=100 rad/s^2  shock_limit=1  report_fault=simscape.enum.assert.action.none  thermal_port=simscape.enum.thermaleffects.omit  thermal_mass=50 kJ/K  temperature_specify=off  temperature_priority=High  temperature=300 K  temperature_nominal_specify=off  temperature_nominal_unit=K  temperature_nominal_value=1
  Simscape Bus : SimscapeBus  HierarchyStrings=AxlFL;AxlFR;AxlRL;AxlRR
  Simscape Bus1 : SimscapeBus  HierarchyStrings=AxlFL;AxlFR;AxlRL;AxlRR
  Simulink-PS Converter{,1..3} (4 alike) : nesl_utility_internal/Simulink-PS Converter  PhysicalDomain=network_engine_domain  SubClassName=ps_input  LeftPortType=input  RightPortType=output  PseudoPeriodic=off  Frequencies=[]  NoiseDistribution=none  NoiseParameters=[]  Unit=1  AffineConversion=off  FilteringAndDerivatives=provide  SimscapeFilterOrder=1  InputFilterTimeConstant=0.001  UdotUserProvided=0
  Solver Configuration : nesl_utility_internal/Solver Configuration  PhysicalDomain=network_engine_domain  SubClassName=solver  LeftPortType=input  RightPortType=generic  Tones=[]  Harmonics=[]  SimulateNoise=off  Profile=off  UseLocalSampling=off  EnableSwitchedLinearOptims=on  FrequencyDomain=off  UseCCode=off  RelTol=0.001  AbsTol=0.001  MinStep=1e-09  ToWorkspace=off  RevertToSquareIcSolve=off  NumHomotopyIterations=100  PhasorMode=off  PhasorModeNumHarmonics=1  ConsistencySolver=NEWTON_XTOL_AFTER_FTOL  IndexReductionMethod=DerivativeReplacement  DoDC=off  ResidualTolerance=1e-09  ConsistencyTolSource=GLOBAL  ConsistencyAbsTol=0.001  ConsistencyRelTol=0.001  ConsistencyTolFactor=0.001  UseLocalSolver=off  LocalSolverChoice=NE_BACKWARD_EULER_ADVANCER  ResolveIndetEquations=on  FunctionEvalNumThread=1  LocalSolverSampleTime=0.001  DoFixedCost=off  MaxNonlinIter=3  MaxModeIter=2  ComputeImpulses=off  ImpulseIterations=2  LinearAlgebra=auto  LinearAlgebraNumThread=0  EquationFormulation=NE_TIME_EF  DelaysMemoryBudget=1024  AutomaticFiltering=on  FilteringTimeConstant=0.001  PartitionStorageMethod=AS_NEEDED  PartitionMemoryBudget=1024  PartitionMethod=ROBUST
  Step : Step  After=100  SampleTime=0
  Step1 : Step  After=100  SampleTime=0
  Vector Concatenate1 : Concatenate  NumInputs=4
  AxlTrqIn : PMIOPort  Side=Left
  AxlTrqOut : PMIOPort  Port=2  Side=Right
  BrkPrsCmdOut : Outport
  wires:
  Constant2/1 -> Vector Concatenate1/1
  Constant3/1 -> Vector Concatenate1/2
  Constant4/1 -> Vector Concatenate1/3
  Vector Concatenate1/1 -> BrkPrsCmdOut/1
  Constant5/1 -> Vector Concatenate1/4
  Step1/1 -> Simulink-PS Converter1/1
  Step/1 -> Simulink-PS Converter/1
  Constant1/1 -> Simulink-PS Converter3/1
  Constant/1 -> Simulink-PS Converter2/1
  connections:
  Rotational Damper/LConn1 -- Simscape Bus1/LConn1 -- Solver Configuration/RConn1
  Rotational Damper2/LConn1 -- Simscape Bus1/LConn3 -- Rotational Damper1/RConn1
  Simscape Bus1/LConn4 -- Rotational Damper2/RConn1 -- Mechanical Rotational Reference7/LConn1
  Rotational Damper1/LConn1 -- Rotational Damper/RConn1 -- Simscape Bus1/LConn2
  Simulink-PS Converter3/RConn1 -- RR1/RConn1
  AxlTrqOut/RConn1 -- Simscape Bus/RConn1
  RR1/LConn1 -- Simscape Bus/LConn4
  Mechanical Rotational Reference1/LConn1 -- FR1/RConn2
  FR1/LConn1 -- Simscape Bus/LConn2
  AxlTrqIn/RConn1 -- Simscape Bus1/RConn1
  Simulink-PS Converter2/RConn1 -- RL1/RConn1
  RL1/LConn1 -- Simscape Bus/LConn3
  Mechanical Rotational Reference/LConn1 -- FL1/RConn2
  Simulink-PS Converter/RConn1 -- FL1/RConn1
  Mechanical Rotational Reference3/LConn1 -- RR1/RConn2
  Simscape Bus/LConn1 -- FL1/LConn1
  Simulink-PS Converter1/RConn1 -- FR1/RConn1
  Mechanical Rotational Reference2/LConn1 -- RL1/RConn2

== system ConfiguredSimscapePlantModels/Body, Suspension, Wheels/Powertrain Bypass/Pass Through ==
  BrkPrsCmdIn : Inport
  AxlTrqIn : PMIOPort  Side=Left
  AxlTrqOut : PMIOPort  Port=2  Side=Right
  BrkPrsCmdOut : Outport
  wires:
  BrkPrsCmdIn/1 -> BrkPrsCmdOut/1
  connections:
  AxlTrqOut/RConn1 -- AxlTrqIn/RConn1

== system ConfiguredSimscapePlantModels/Drivetrain/Drivetrain Layout/AxlTrqFL ==
  Ideal Torque Sensor : fl_lib/Mechanical/Mechanical Sensors/Ideal Torque Sensor
  PS-Simulink Converter : nesl_utility_internal/PS-Simulink Converter  PhysicalDomain=network_engine_domain  SubClassName=ps_output  LeftPortType=input  RightPortType=output  PseudoPeriodic=off  Frequencies=[]  VectorFormat=inherit  Unit=inherit  AffineConversion=off
  R : PMIOPort  Side=Left
  C : PMIOPort  Port=2  Side=Right
  Trq : Outport
  wires:
  PS-Simulink Converter/1 -> Trq/1
  connections:
  Ideal Torque Sensor/LConn1 -- R/RConn1
  Ideal Torque Sensor/RConn1 -- C/RConn1
  PS-Simulink Converter/LConn1 -- Ideal Torque Sensor/RConn2

== system ConfiguredSimscapePlantModels/Drivetrain/Drivetrain Layout/AxlTrqFR ==
  Ideal Torque Sensor : fl_lib/Mechanical/Mechanical Sensors/Ideal Torque Sensor
  PS-Simulink Converter : nesl_utility_internal/PS-Simulink Converter  PhysicalDomain=network_engine_domain  SubClassName=ps_output  LeftPortType=input  RightPortType=output  PseudoPeriodic=off  Frequencies=[]  VectorFormat=inherit  Unit=inherit  AffineConversion=off
  R : PMIOPort  Side=Left
  C : PMIOPort  Port=2  Side=Right
  Trq : Outport
  wires:
  PS-Simulink Converter/1 -> Trq/1
  connections:
  PS-Simulink Converter/LConn1 -- Ideal Torque Sensor/RConn2
  Ideal Torque Sensor/RConn1 -- C/RConn1
  Ideal Torque Sensor/LConn1 -- R/RConn1

== system ConfiguredSimscapePlantModels/Drivetrain/Drivetrain Layout/AxlTrqR ==
  Ideal Torque Sensor : fl_lib/Mechanical/Mechanical Sensors/Ideal Torque Sensor
  PS-Simulink Converter : nesl_utility_internal/PS-Simulink Converter  PhysicalDomain=network_engine_domain  SubClassName=ps_output  LeftPortType=input  RightPortType=output  PseudoPeriodic=off  Frequencies=[]  VectorFormat=inherit  Unit=inherit  AffineConversion=off
  R : PMIOPort  Side=Left
  C : PMIOPort  Port=2  Side=Right
  Trq : Outport
  wires:
  PS-Simulink Converter/1 -> Trq/1
  connections:
  PS-Simulink Converter/LConn1 -- Ideal Torque Sensor/RConn2
  Ideal Torque Sensor/RConn1 -- C/RConn1
  Ideal Torque Sensor/LConn1 -- R/RConn1

== system ConfiguredSimscapePlantModels/Drivetrain/Drivetrain Layout/AxlTrqRL ==
  Ideal Torque Sensor : fl_lib/Mechanical/Mechanical Sensors/Ideal Torque Sensor
  PS-Simulink Converter : nesl_utility_internal/PS-Simulink Converter  PhysicalDomain=network_engine_domain  SubClassName=ps_output  LeftPortType=input  RightPortType=output  PseudoPeriodic=off  Frequencies=[]  VectorFormat=inherit  Unit=inherit  AffineConversion=off
  R : PMIOPort  Side=Left
  C : PMIOPort  Port=2  Side=Right
  Trq : Outport
  wires:
  PS-Simulink Converter/1 -> Trq/1
  connections:
  Ideal Torque Sensor/LConn1 -- R/RConn1
  Ideal Torque Sensor/RConn1 -- C/RConn1
  PS-Simulink Converter/LConn1 -- Ideal Torque Sensor/RConn2

== system ConfiguredSimscapePlantModels/Drivetrain/Drivetrain Layout/Axle Interconnect ==
  SplitRatio : Inport
  Lockup : Inport  Port=2
  No Interconnect : Subsystem  VariantControl=No Interconnect
  FrntDiffrntlTrq : PMIOPort  Side=Left
  DriveshftTrq : PMIOPort  Port=2  Side=Left
  RearDiffrntlTrq : PMIOPort  Port=3  Side=Left

== system ConfiguredSimscapePlantModels/Drivetrain/Drivetrain Layout/DriveshftTrq Routing ==
  One Actuator FWD : Subsystem  VariantControl=One Actuator FWD  ReferencedSubsystem=OneActuatorFWDSSC
  Two Actuator AWD : Subsystem  VariantControl=Two Actuator AWD  ReferencedSubsystem=OneActuatorFWDSSC
  DriveshftTrq : PMIOPort  Side=Left
  FrntDiffrntlTrq : PMIOPort  Port=2  Side=Right
  TrnsfrCaseFrntTrq : PMIOPort  Port=3  Side=Right
  TrnsfrCaseTrq : PMIOPort  Port=4  Side=Right
  TrnsfrCaseRearTrq : PMIOPort  Port=5  Side=Right
  RearDiffrntlTrq : PMIOPort  Port=6  Side=Right
  DriveshftSpd : Outport  VectorParamsAs1DForOutWhenUnconnected=off

== system ConfiguredSimscapePlantModels/Drivetrain/Drivetrain Layout/Front Axle ==
  Prs1 : Inport
  Prs2 : Inport  Port=2
  Open Differential : Subsystem  VariantControl=Open Differential  ReferencedSubsystem=OpenDifferentialSSC
  Open Differential with Loss : Subsystem  VariantControl=Loss
  DriveshftTrq : PMIOPort  Side=Left
  AxlTrqFL : PMIOPort  Port=2  Side=Right
  AxlTrqFR : PMIOPort  Port=3  Side=Right
  Info : Outport
  DriveshftSpd : Outport  Port=2
  Axl1Spd : Outport  Port=3
  Axl2Spd : Outport  Port=4

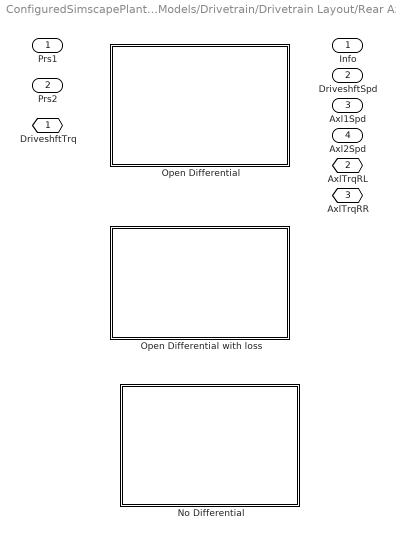
== system ConfiguredSimscapePlantModels/Drivetrain/Drivetrain Layout/Rear Axle ==
  Prs1 : Inport
  Prs2 : Inport  Port=2
  No Differential : Subsystem  VariantControl=No Differential  ReferencedSubsystem=NoDifferentialRearSSC
  Open Differential : Subsystem  VariantControl=Open Differential  ReferencedSubsystem=OpenDifferential2SSC
  Open Differential with loss : Subsystem  VariantControl=Loss
  DriveshftTrq : PMIOPort  Side=Left
  AxlTrqRL : PMIOPort  Port=2  Side=Right
  AxlTrqRR : PMIOPort  Port=3  Side=Right
  Info : Outport
  DriveshftSpd : Outport  Port=2
  Axl1Spd : Outport  Port=3
  Axl2Spd : Outport  Port=4

== system ConfiguredSimscapePlantModels/Electrical System/Electrical System 1EM/Battery System ==
  note: 1) Add Subsystem or Model blocks as valid variant choices.
      | 2) You cannot connect blocks at this level. At simulation, connectivity is automatically
      | determined, based on the active variant and port name matching.
  P_Acc : Inport
  BMS : Inport  Port=2
  AmbTemp : Inport  Port=3
  Mapped Battery : Subsystem  VariantControl=Mapped Battery  ReferencedSubsystem=BatteryMappedSSC
  + : PMIOPort  Side=Right
  - : PMIOPort  Port=2  Side=Right
  BattSoc : Outport  VectorParamsAs1DForOutWhenUnconnected=off
  BattVolt : Outport  Port=2  VectorParamsAs1DForOutWhenUnconnected=off
  BattCurr : Outport  Port=3  VectorParamsAs1DForOutWhenUnconnected=off
  BMSSensors : Outport  Port=4  VectorParamsAs1DForOutWhenUnconnected=off

== system ConfiguredSimscapePlantModels/Electrical System/Electrical System 1EM/DC-DC Converter ==
  DC-DC Converter : Subsystem  VariantControl=DC-DC Converter  ReferencedSubsystem=DCDCConverterSSC
  No DC-DC Converter : Subsystem  VariantControl=No DC-DC Converter
  1+ : PMIOPort  Side=Left
  2+ : PMIOPort  Port=2  Side=Right
  1- : PMIOPort  Port=3  Side=Left
  2- : PMIOPort  Port=4  Side=Right
  H : PMIOPort  Port=5  Side=Right
  Vref : PMIOPort  Port=6  Side=Left

== system ConfiguredSimscapePlantModels/Electrical System/Electrical System 1EM/Front EM ==
  EMTrqCmd : Inport
  + : PMIOPort  Side=Left
  - : PMIOPort  Port=2  Side=Left
  R : PMIOPort  Port=3  Side=Right
  EMTrq : Outport  VectorParamsAs1DForOutWhenUnconnected=off
  EMPwrElec : Outport  Port=2
  EMPwrMech : Outport  Port=3

== system ConfiguredSimscapePlantModels/Electrical System/Electrical System 1EM/Rear EM ==
  EMTrqCmd : Inport
  + : PMIOPort  Side=Left
  - : PMIOPort  Port=2  Side=Left
  R : PMIOPort  Port=3  Side=Right
  EMTrq : Outport  VectorParamsAs1DForOutWhenUnconnected=off
  EMPwrElec : Outport  Port=2
  EMPwrMech : Outport  Port=3

== system ConfiguredSimscapePlantModels/Sensors/Sensors/No IMU Sensor ==
  VehFdbk : Inport
  Bus Creator1 : BusCreator  Inputs=2
  Constant : Constant  Value=zeros(3,1)
  Constant1 : Constant  Value=zeros(3,1)
  Terminator : Terminator
  IMU : Outport
  wires:
  VehFdbk/1 -> Terminator/1
  Constant1/1 -> Bus Creator1/2  "pqr"
  Bus Creator1/1 -> IMU/1  "IMU"
  Constant/1 -> Bus Creator1/1  "Acc"

== system ConfiguredSimscapePlantModels/Drivetrain/Drivetrain Layout/Axle Interconnect/No Interconnect ==
